simulink model "Ejemplo02"  (R2021b)
settings: Solver=VariableStepAuto  StartTime=2  StopTime=10  RelTol=1e-3
settings Model: Creator=juandiegocastropadilla  LastModifiedBy=juandiegocastropadilla

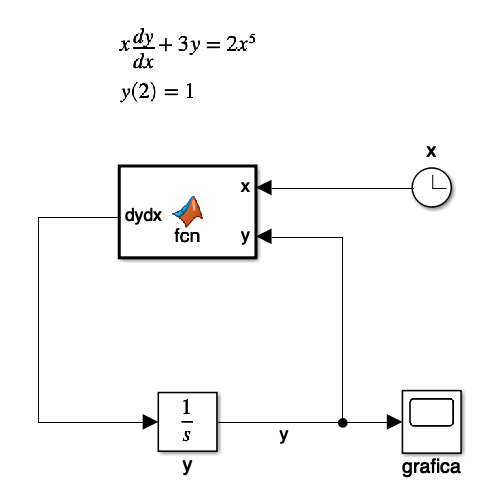
[thumbnail: Simulink's stored preview of the top-level diagram]
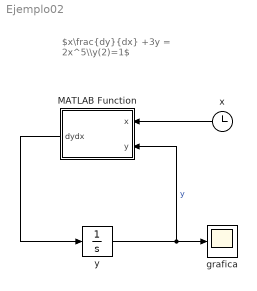
== system Ejemplo02 ==
  note: $x\frac{dy}{dx} +3y = 2x^5\\y(2)=1$
  MATLAB Function : MATLAB Function  TreatAsAtomicUnit=on
  grafica : Scope
  x : Clock
  y : Integrator  InitialCondition=1
  wires:
  MATLAB Function/1(dydx) -> y/1
  y/1 -> MATLAB Function/2(y), grafica/1  "y"
  x/1 -> MATLAB Function/1(x)

== matlab function Ejemplo02/MATLAB Function ==
  data: x input; y input; dydx output
function dydx = fcn(x, y)

dydx = (2*x^5 - 3*y)/x;
